simulink model "Pokus01_JK_Latch"  (Simulink 8.1)
settings: Solver=ode45  StartTime=0.0  StopTime=5.0  RelTol=1e-3
libraries: simulink_extras x4
settings Model: Creator=uzivatel  LastModifiedBy=uzivatel
settings DataIOCC: SignalLoggingSaveFormat=Dataset
settings OptimizationCC: ExpressionDepthLimit=128
settings DebuggingCC: FcnCallInpInsideContextMsg=EnableAllAsError
settings GRTTargetCC: CombineOutputUpdateFcns=on  GRTInterface=off

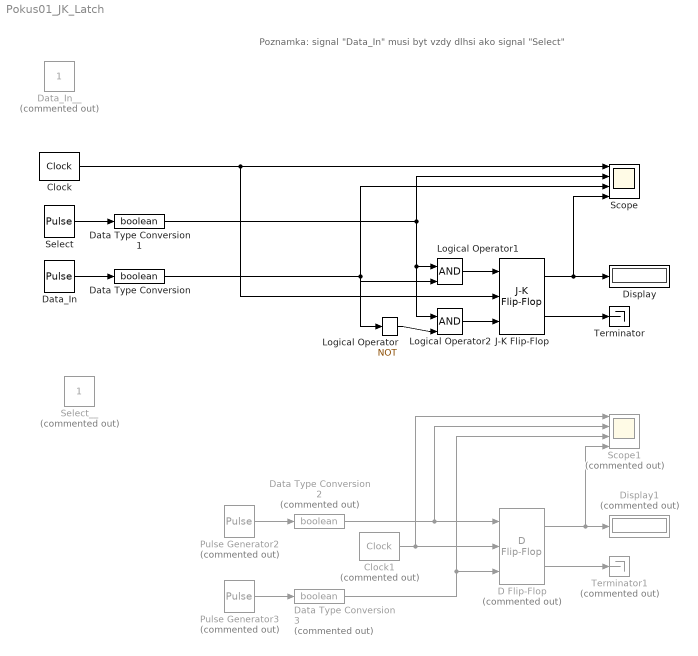
== system Pokus01_JK_Latch ==
  note: Poznamka: signal "Data_In" musi byt vzdy dlhsi ako signal "Select"
  Clock : simulink_extras/Flip Flops/Clock  period=1
  Clock1 : simulink_extras/Flip Flops/Clock  Commented=on  period=1
  D Flip-Flop : simulink_extras/Flip Flops/D Flip-Flop  Commented=on
  Data Type Conversion : DataTypeConversion  OutDataTypeStr=boolean
  Data Type Conversion1 : DataTypeConversion  OutDataTypeStr=boolean
  Data Type Conversion2 : DataTypeConversion  Commented=on  OutDataTypeStr=boolean
  Data Type Conversion3 : DataTypeConversion  Commented=on  OutDataTypeStr=boolean
  Data_In : DiscretePulseGenerator  PulseType=Time based  Period=5  PulseWidth=40  PhaseDelay=0.25
  Data_In__ : Constant  Commented=on
  Display : Display
  Display1 : Display  Commented=on
  J-K Flip-Flop : simulink_extras/Flip Flops/J-K Flip-Flop  initial_condition=0
  Logical Operator : Logic  Operator=NOT  IconShape=distinctive  AllPortsSameDT=off  OutDataTypeStr=boolean
  Logical Operator1 : Logic  IconShape=distinctive  AllPortsSameDT=off  OutDataTypeStr=boolean
  Logical Operator2 : Logic  IconShape=distinctive  AllPortsSameDT=off  OutDataTypeStr=boolean
  Pulse Generator2 : DiscretePulseGenerator  Commented=on  PulseType=Time based  Period=5  PulseWidth=50  PhaseDelay=0.5
  Pulse Generator3 : DiscretePulseGenerator  Commented=on  PulseType=Time based  Period=5  PulseWidth=30  PhaseDelay=0.75
  Scope : Scope  NumInputPorts=4
      settings: YMin=0~0~0~0  YMax=1.5~1.5~1.5~1.5
  Scope1 : Scope  Commented=on  NumInputPorts=4
      settings: YMin=-0.5~-0.5~-0.5~-0.5  YMax=1.5~1.5~1.5~1.5
  Select : DiscretePulseGenerator  PulseType=Time based  Period=3  PulseWidth=10  PhaseDelay=0.25
  Select__ : Constant  Commented=on
  Terminator : Terminator
  Terminator1 : Terminator  Commented=on
  wires:
  J-K Flip-Flop/1 -> Scope/4, Display/1
  J-K Flip-Flop/2 -> Terminator/1
  Clock/1 -> J-K Flip-Flop/2, Scope/1
  Data Type Conversion/1 -> Scope/3, Logical Operator/1, Logical Operator1/2
  Data_In/1 -> Data Type Conversion/1
  Select/1 -> Data Type Conversion1/1
  D Flip-Flop/1 -> Scope1/4, Display1/1
  D Flip-Flop/2 -> Terminator1/1
  Clock1/1 -> D Flip-Flop/2, Scope1/1
  Data Type Conversion2/1 -> D Flip-Flop/1, Scope1/2
  Pulse Generator2/1 -> Data Type Conversion2/1
  Data Type Conversion3/1 -> D Flip-Flop/3, Scope1/3
  Pulse Generator3/1 -> Data Type Conversion3/1
  Logical Operator2/1 -> J-K Flip-Flop/3
  Data Type Conversion1/1 -> Logical Operator2/1, Logical Operator1/1, Scope/2
  Logical Operator1/1 -> J-K Flip-Flop/1
  Logical Operator/1 -> Logical Operator2/2
